simulink model "LQR"  (R2019a)
settings: Solver=FixedStepAuto  StartTime=0.0  StopTime=3  FixedStep=0.0001  RelTol=1e-3
values from neighbouring files (symbols this model uses):
  Cf = 30989    [LQR_Setup.m]
  Cr = 50154    [LQR_Setup.m]
  Iz = 111.8    [LQR_Setup.m]
  lf = 0.783    [LQR_Setup.m]
  lr = 0.752    [LQR_Setup.m]
  m = 245    [LQR_Setup.m]
undefined symbols (not defined in the file or in its folder): DiscIntNeverNeededParam, K1, K2, K3
settings Model: Creator=Johan PC  LastModifiedBy=Johan PC
settings DataIOCC: ReturnWorkspaceOutputs=off
settings DebuggingCC: ArithmeticOperatorsInVariantConditions=warning

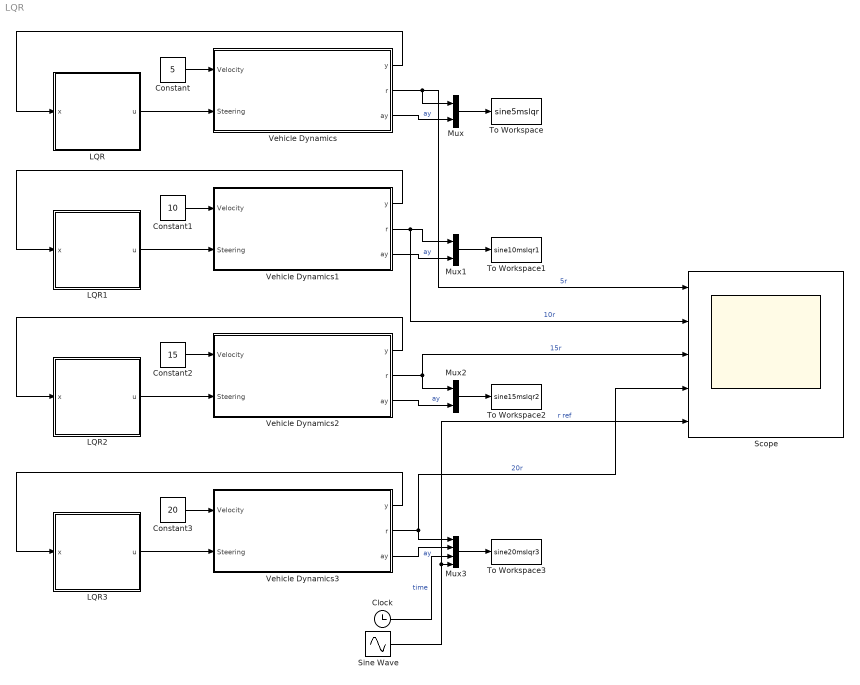
== system LQR ==
  Clock : Clock
  Constant : Constant  Value=5
  Constant1 : Constant  Value=10
  Constant2 : Constant  Value=15
  Constant3 : Constant  Value=20
  LQR : Subsystem
  LQR1 : Subsystem
  LQR2 : Subsystem
  LQR3 : Subsystem
  Mux : Mux  Inputs=2
  Mux1 : Mux  Inputs=2
  Mux2 : Mux  Inputs=2
  Mux3 : Mux
  Scope : Scope  NumInputPorts=5
  Sine Wave : Sin  Amplitude=2  Frequency=2  SampleTime=0
  To Workspace : ToWorkspace  VariableName=sine5mslqr  SampleTime=-1
      settings: Save2DSignal=2-D array (concatenate along first dimension)
  To Workspace1 : ToWorkspace  VariableName=sine10mslqr1  SampleTime=-1
      settings: Save2DSignal=2-D array (concatenate along first dimension)
  To Workspace2 : ToWorkspace  VariableName=sine15mslqr2  SampleTime=-1
      settings: Save2DSignal=2-D array (concatenate along first dimension)
  To Workspace3 : ToWorkspace  VariableName=sine20mslqr3  SampleTime=-1
      settings: Save2DSignal=2-D array (concatenate along first dimension)
  Vehicle Dynamics : Subsystem
  Vehicle Dynamics1 : Subsystem
  Vehicle Dynamics2 : Subsystem
  Vehicle Dynamics3 : Subsystem
  wires:
  Vehicle Dynamics/1("y ") -> LQR/1(x)
  LQR/1(u) -> Vehicle Dynamics/2(Steering)
  Constant/1 -> Vehicle Dynamics/1(Velocity)
  Vehicle Dynamics/2("r ") -> Scope/1, Mux/1  "5r"
  Vehicle Dynamics/3(ay) -> Mux/2  "ay"
  Mux/1 -> To Workspace/1
  Constant1/1 -> Vehicle Dynamics1/1(Velocity)
  Vehicle Dynamics1/1("y ") -> LQR1/1(x)
  LQR1/1(u) -> Vehicle Dynamics1/2(Steering)
  Vehicle Dynamics1/2("r ") -> Scope/2, Mux1/1  "10r"
  Vehicle Dynamics1/3(ay) -> Mux1/2  "ay"
  Mux1/1 -> To Workspace1/1
  Constant2/1 -> Vehicle Dynamics2/1(Velocity)
  Vehicle Dynamics2/1("y ") -> LQR2/1(x)
  LQR2/1(u) -> Vehicle Dynamics2/2(Steering)
  Vehicle Dynamics2/2("r ") -> Mux2/1, Scope/3  "15r"
  Vehicle Dynamics2/3(ay) -> Mux2/2  "ay"
  Mux2/1 -> To Workspace2/1
  Constant3/1 -> Vehicle Dynamics3/1(Velocity)
  Vehicle Dynamics3/1("y ") -> LQR3/1(x)
  LQR3/1(u) -> Vehicle Dynamics3/2(Steering)
  Vehicle Dynamics3/2("r ") -> Mux3/1, Scope/4  "20r"
  Vehicle Dynamics3/3(ay) -> Mux3/2  "ay"
  Mux3/1 -> To Workspace3/1
  Clock/1 -> Mux3/3  "time"
  Sine Wave/1 -> Scope/5, Mux3/4  "r ref"

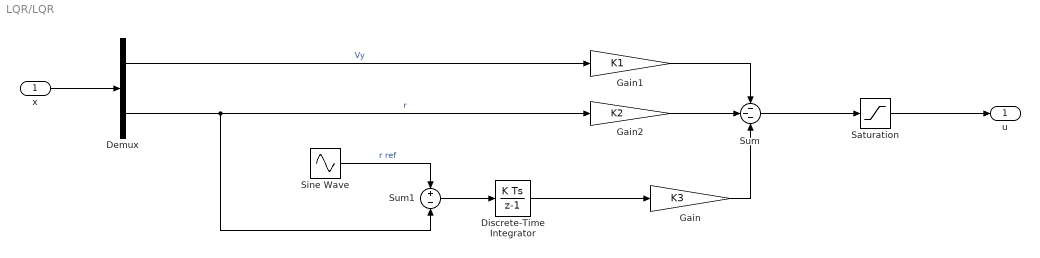
== system LQR/LQR ==
  x : Inport
  Demux : Demux  Outputs=2
  Discrete-Time Integrator : DiscreteIntegrator  SampleTime=0.001  ICPrevOutput=DiscIntNeverNeededParam  ICPrevScaledInput=DiscIntNeverNeededParam
  Gain : Gain  Gain=K3
  Gain1 : Gain  Gain=K1
  Gain2 : Gain  Gain=K2
  Saturation : Saturate  UpperLimit=0.45  LowerLimit=-0.45
  Sine Wave : Sin  Amplitude=2  Frequency=2  SampleTime=0
  Sum : Sum  Inputs=---
  Sum1 : Sum  Inputs=+-
  u : Outport
  wires:
  Discrete-Time Integrator/1 -> Gain/1
  Gain/1 -> Sum/3
  x/1 -> Demux/1
  Demux/1 -> Gain1/1  "Vy"
  Demux/2 -> Gain2/1, Sum1/2  "r"
  Gain1/1 -> Sum/1
  Gain2/1 -> Sum/2
  Sum/1 -> Saturation/1
  Sum1/1 -> Discrete-Time Integrator/1
  Sine Wave/1 -> Sum1/1  "r ref"
  Saturation/1 -> u/1

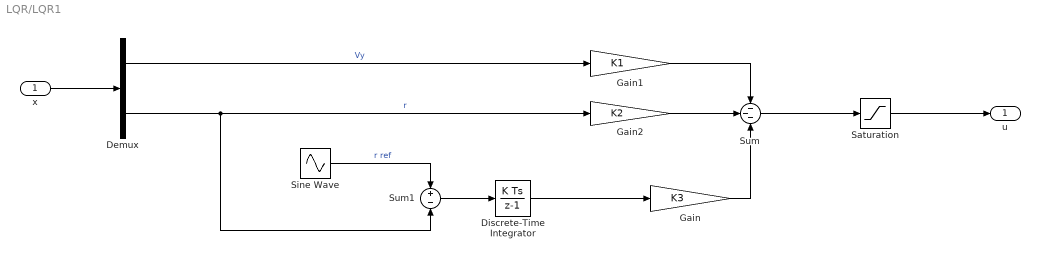
== system LQR/LQR1 ==
  x : Inport
  Demux : Demux  Outputs=2
  Discrete-Time Integrator : DiscreteIntegrator  SampleTime=0.001  ICPrevOutput=DiscIntNeverNeededParam  ICPrevScaledInput=DiscIntNeverNeededParam
  Gain : Gain  Gain=K3
  Gain1 : Gain  Gain=K1
  Gain2 : Gain  Gain=K2
  Saturation : Saturate  UpperLimit=0.45  LowerLimit=-0.45
  Sine Wave : Sin  Amplitude=2  Frequency=2  SampleTime=0
  Sum : Sum  Inputs=---
  Sum1 : Sum  Inputs=+-
  u : Outport
  wires:
  Discrete-Time Integrator/1 -> Gain/1
  Gain/1 -> Sum/3
  x/1 -> Demux/1
  Demux/1 -> Gain1/1  "Vy"
  Demux/2 -> Gain2/1, Sum1/2  "r"
  Gain1/1 -> Sum/1
  Gain2/1 -> Sum/2
  Sum/1 -> Saturation/1
  Sum1/1 -> Discrete-Time Integrator/1
  Sine Wave/1 -> Sum1/1  "r ref"
  Saturation/1 -> u/1

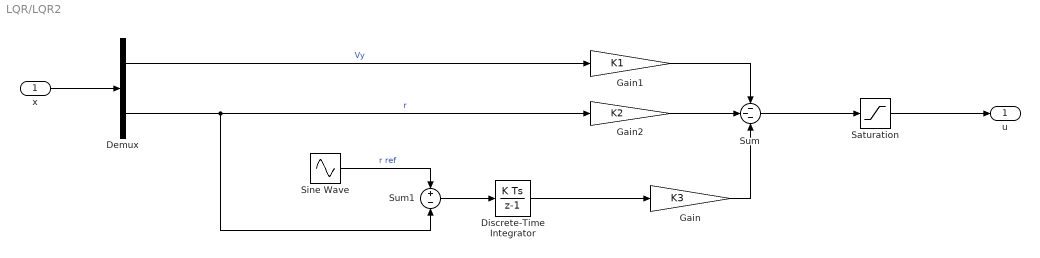
== system LQR/LQR2 ==
  x : Inport
  Demux : Demux  Outputs=2
  Discrete-Time Integrator : DiscreteIntegrator  SampleTime=0.001  ICPrevOutput=DiscIntNeverNeededParam  ICPrevScaledInput=DiscIntNeverNeededParam
  Gain : Gain  Gain=K3
  Gain1 : Gain  Gain=K1
  Gain2 : Gain  Gain=K2
  Saturation : Saturate  UpperLimit=0.45  LowerLimit=-0.45
  Sine Wave : Sin  Amplitude=2  Frequency=2  SampleTime=0
  Sum : Sum  Inputs=---
  Sum1 : Sum  Inputs=+-
  u : Outport
  wires:
  Discrete-Time Integrator/1 -> Gain/1
  Gain/1 -> Sum/3
  x/1 -> Demux/1
  Demux/1 -> Gain1/1  "Vy"
  Demux/2 -> Gain2/1, Sum1/2  "r"
  Gain1/1 -> Sum/1
  Gain2/1 -> Sum/2
  Sum/1 -> Saturation/1
  Sum1/1 -> Discrete-Time Integrator/1
  Sine Wave/1 -> Sum1/1  "r ref"
  Saturation/1 -> u/1

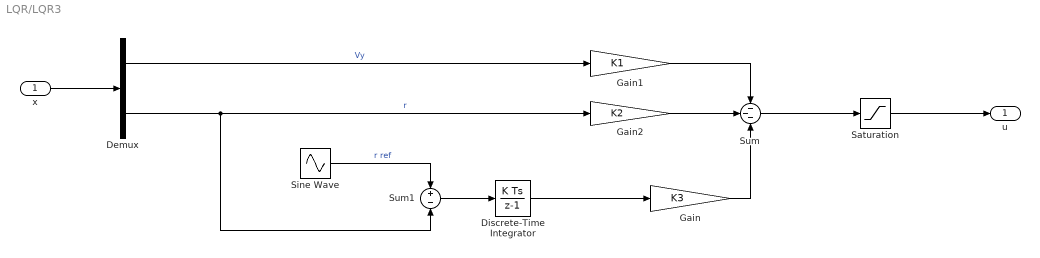
== system LQR/LQR3 ==
  x : Inport
  Demux : Demux  Outputs=2
  Discrete-Time Integrator : DiscreteIntegrator  SampleTime=0.001  ICPrevOutput=DiscIntNeverNeededParam  ICPrevScaledInput=DiscIntNeverNeededParam
  Gain : Gain  Gain=K3
  Gain1 : Gain  Gain=K1
  Gain2 : Gain  Gain=K2
  Saturation : Saturate  UpperLimit=0.45  LowerLimit=-0.45
  Sine Wave : Sin  Amplitude=2  Frequency=2  SampleTime=0
  Sum : Sum  Inputs=---
  Sum1 : Sum  Inputs=+-
  u : Outport
  wires:
  Discrete-Time Integrator/1 -> Gain/1
  Gain/1 -> Sum/3
  x/1 -> Demux/1
  Demux/1 -> Gain1/1  "Vy"
  Demux/2 -> Gain2/1, Sum1/2  "r"
  Gain1/1 -> Sum/1
  Gain2/1 -> Sum/2
  Sum/1 -> Saturation/1
  Sum1/1 -> Discrete-Time Integrator/1
  Sine Wave/1 -> Sum1/1  "r ref"
  Saturation/1 -> u/1

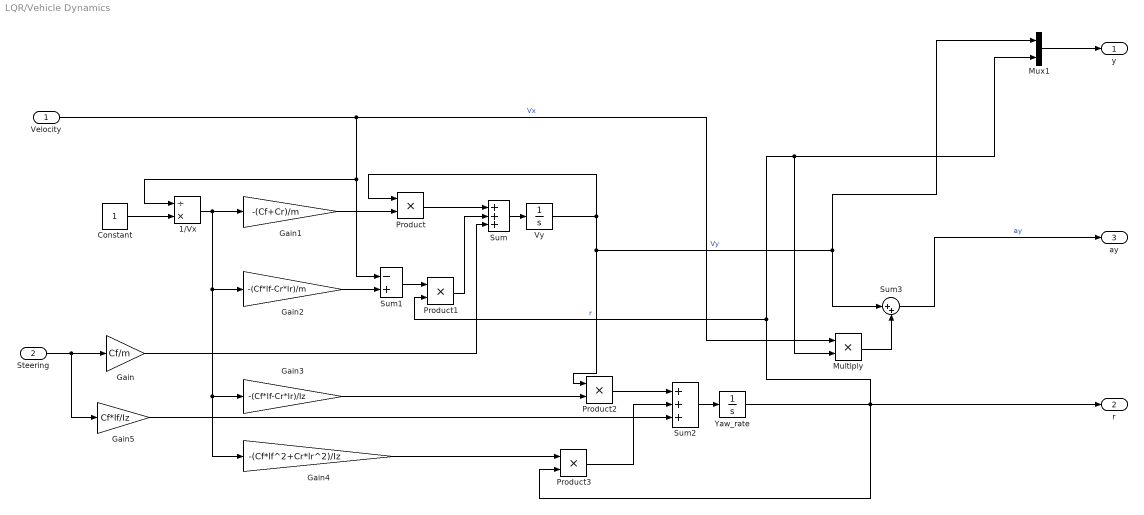
== system LQR/Vehicle Dynamics ==
  Velocity : Inport
  Steering : Inport  Port=2
  1/Vx : Product  Inputs=/*
  Constant : Constant
  Gain : Gain  Gain=Cf/m
  Gain1 : Gain  Gain=-(Cf+Cr)/m
  Gain2 : Gain  Gain=-(Cf*lf-Cr*lr)/m
  Gain3 : Gain  Gain=-(Cf*lf-Cr*lr)/Iz
  Gain4 : Gain  Gain=-(Cf*lf^2+Cr*lr^2)/Iz
  Gain5 : Gain  Gain=Cf*lf/Iz
  Multiply : Product
  Mux1 : Mux  Inputs=2
  Product{,1..3} (4 alike) : Product
  Sum : Sum  Inputs=+++
  Sum1 : Sum  Inputs=-+
  Sum2 : Sum  Inputs=+++
  Sum3 : Sum  Inputs=|++
  Vy : Integrator
  "Yaw_rate " : Integrator
  "y " : Outport
  "r " : Outport  Port=2
  ay : Outport  Port=3
  wires:
  Sum2/1 -> "Yaw_rate "/1
  Gain2/1 -> Sum1/2
  Gain4/1 -> Product3/1
  Constant/1 -> 1/Vx/2
  Gain3/1 -> Product2/2
  1/Vx/1 -> Gain4/1, Gain3/1, Gain2/1, Gain1/1
  Product2/1 -> Sum2/1
  Product3/1 -> Sum2/2
  Gain5/1 -> Sum2/3
  Sum1/1 -> Product1/1
  "Yaw_rate "/1 -> Multiply/2, Mux1/2, Product1/2, "r "/1, Product3/2  "r"
  Gain/1 -> Sum/3
  Steering/1 -> Gain/1, Gain5/1
  Gain1/1 -> Product/2
  Product/1 -> Sum/1
  Vy/1 -> Mux1/1, Sum3/1, Product2/1, Product/1  "Vy"
  Sum/1 -> Vy/1
  Velocity/1 -> Multiply/1, 1/Vx/1, Sum1/1  "Vx"
  Product1/1 -> Sum/2
  Multiply/1 -> Sum3/2
  Sum3/1 -> ay/1  "ay"
  Mux1/1 -> "y "/1

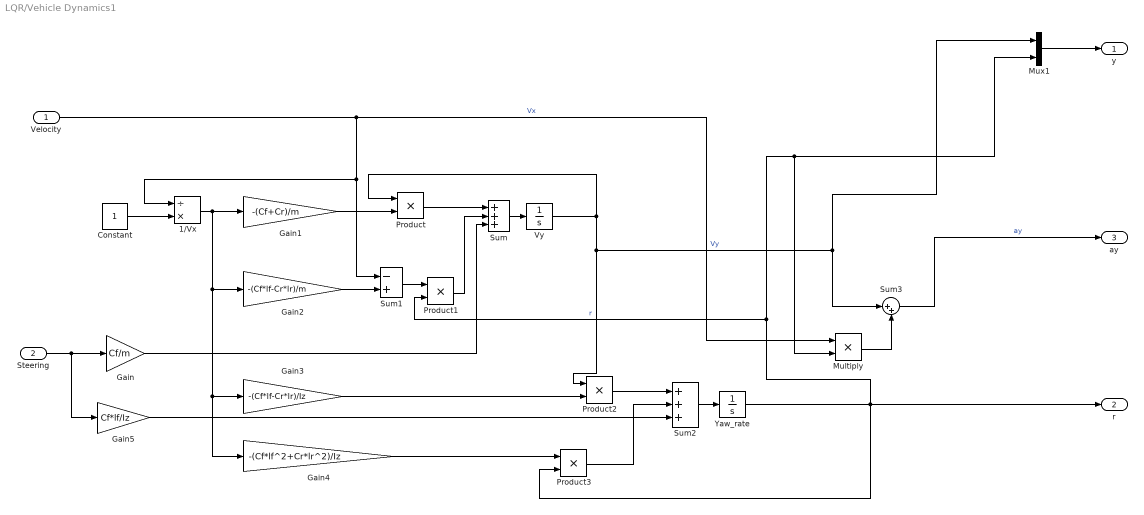
== system LQR/Vehicle Dynamics1 ==
  Velocity : Inport
  Steering : Inport  Port=2
  1/Vx : Product  Inputs=/*
  Constant : Constant
  Gain : Gain  Gain=Cf/m
  Gain1 : Gain  Gain=-(Cf+Cr)/m
  Gain2 : Gain  Gain=-(Cf*lf-Cr*lr)/m
  Gain3 : Gain  Gain=-(Cf*lf-Cr*lr)/Iz
  Gain4 : Gain  Gain=-(Cf*lf^2+Cr*lr^2)/Iz
  Gain5 : Gain  Gain=Cf*lf/Iz
  Multiply : Product
  Mux1 : Mux  Inputs=2
  Product{,1..3} (4 alike) : Product
  Sum : Sum  Inputs=+++
  Sum1 : Sum  Inputs=-+
  Sum2 : Sum  Inputs=+++
  Sum3 : Sum  Inputs=|++
  Vy : Integrator
  "Yaw_rate " : Integrator
  "y " : Outport
  "r " : Outport  Port=2
  ay : Outport  Port=3
  wires:
  Sum2/1 -> "Yaw_rate "/1
  Gain2/1 -> Sum1/2
  Gain4/1 -> Product3/1
  Constant/1 -> 1/Vx/2
  Gain3/1 -> Product2/2
  1/Vx/1 -> Gain4/1, Gain3/1, Gain2/1, Gain1/1
  Product2/1 -> Sum2/1
  Product3/1 -> Sum2/2
  Gain5/1 -> Sum2/3
  Sum1/1 -> Product1/1
  "Yaw_rate "/1 -> Multiply/2, Mux1/2, Product1/2, "r "/1, Product3/2  "r"
  Gain/1 -> Sum/3
  Steering/1 -> Gain/1, Gain5/1
  Gain1/1 -> Product/2
  Product/1 -> Sum/1
  Vy/1 -> Mux1/1, Sum3/1, Product2/1, Product/1  "Vy"
  Sum/1 -> Vy/1
  Velocity/1 -> Multiply/1, 1/Vx/1, Sum1/1  "Vx"
  Product1/1 -> Sum/2
  Multiply/1 -> Sum3/2
  Sum3/1 -> ay/1  "ay"
  Mux1/1 -> "y "/1

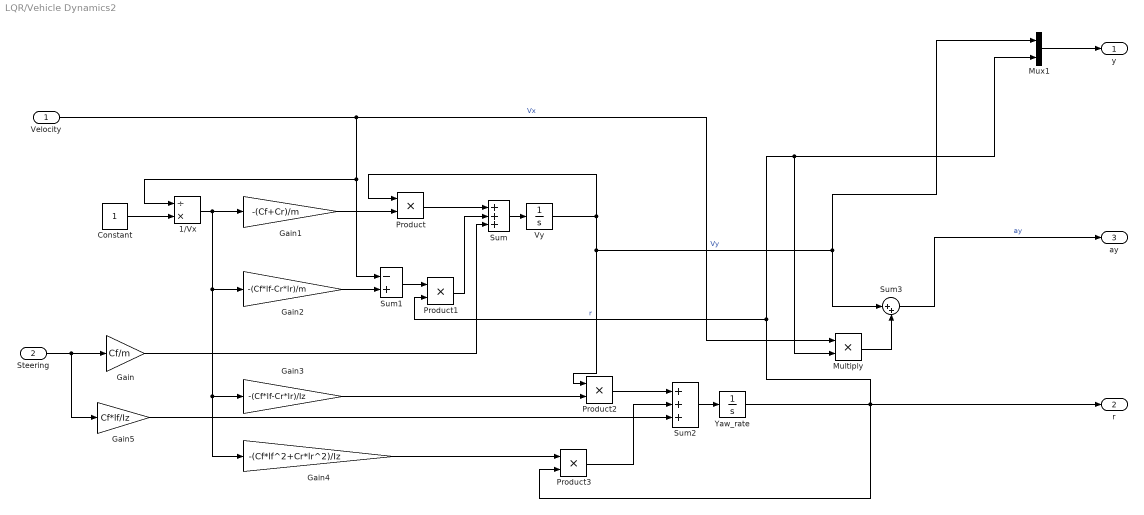
== system LQR/Vehicle Dynamics2 ==
  Velocity : Inport
  Steering : Inport  Port=2
  1/Vx : Product  Inputs=/*
  Constant : Constant
  Gain : Gain  Gain=Cf/m
  Gain1 : Gain  Gain=-(Cf+Cr)/m
  Gain2 : Gain  Gain=-(Cf*lf-Cr*lr)/m
  Gain3 : Gain  Gain=-(Cf*lf-Cr*lr)/Iz
  Gain4 : Gain  Gain=-(Cf*lf^2+Cr*lr^2)/Iz
  Gain5 : Gain  Gain=Cf*lf/Iz
  Multiply : Product
  Mux1 : Mux  Inputs=2
  Product{,1..3} (4 alike) : Product
  Sum : Sum  Inputs=+++
  Sum1 : Sum  Inputs=-+
  Sum2 : Sum  Inputs=+++
  Sum3 : Sum  Inputs=|++
  Vy : Integrator
  "Yaw_rate " : Integrator
  "y " : Outport
  "r " : Outport  Port=2
  ay : Outport  Port=3
  wires:
  Sum2/1 -> "Yaw_rate "/1
  Gain2/1 -> Sum1/2
  Gain4/1 -> Product3/1
  Constant/1 -> 1/Vx/2
  Gain3/1 -> Product2/2
  1/Vx/1 -> Gain4/1, Gain3/1, Gain2/1, Gain1/1
  Product2/1 -> Sum2/1
  Product3/1 -> Sum2/2
  Gain5/1 -> Sum2/3
  Sum1/1 -> Product1/1
  "Yaw_rate "/1 -> Multiply/2, Mux1/2, Product1/2, "r "/1, Product3/2  "r"
  Gain/1 -> Sum/3
  Steering/1 -> Gain/1, Gain5/1
  Gain1/1 -> Product/2
  Product/1 -> Sum/1
  Vy/1 -> Mux1/1, Sum3/1, Product2/1, Product/1  "Vy"
  Sum/1 -> Vy/1
  Velocity/1 -> Multiply/1, 1/Vx/1, Sum1/1  "Vx"
  Product1/1 -> Sum/2
  Multiply/1 -> Sum3/2
  Sum3/1 -> ay/1  "ay"
  Mux1/1 -> "y "/1

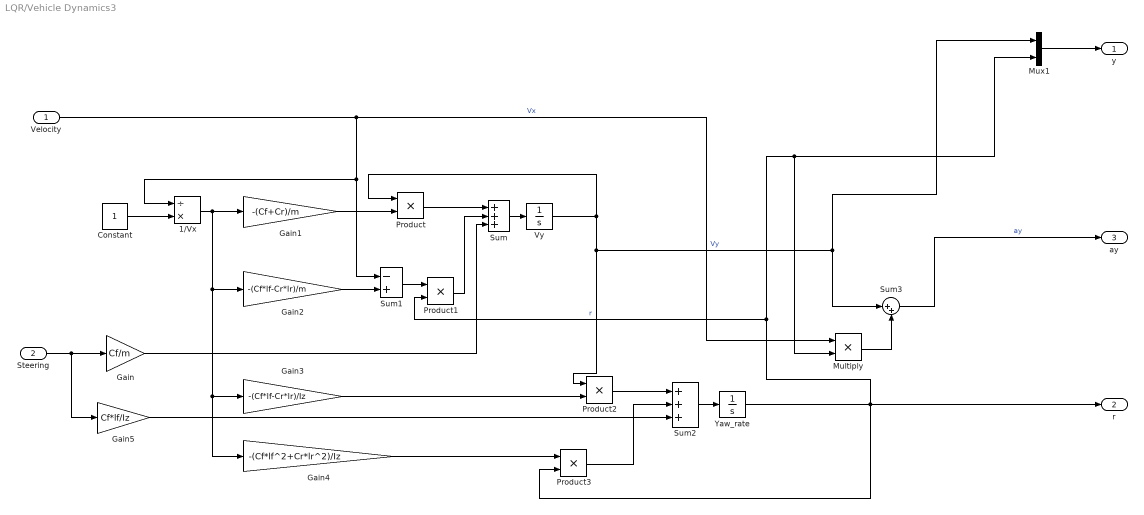
== system LQR/Vehicle Dynamics3 ==
  Velocity : Inport
  Steering : Inport  Port=2
  1/Vx : Product  Inputs=/*
  Constant : Constant
  Gain : Gain  Gain=Cf/m
  Gain1 : Gain  Gain=-(Cf+Cr)/m
  Gain2 : Gain  Gain=-(Cf*lf-Cr*lr)/m
  Gain3 : Gain  Gain=-(Cf*lf-Cr*lr)/Iz
  Gain4 : Gain  Gain=-(Cf*lf^2+Cr*lr^2)/Iz
  Gain5 : Gain  Gain=Cf*lf/Iz
  Multiply : Product
  Mux1 : Mux  Inputs=2
  Product{,1..3} (4 alike) : Product
  Sum : Sum  Inputs=+++
  Sum1 : Sum  Inputs=-+
  Sum2 : Sum  Inputs=+++
  Sum3 : Sum  Inputs=|++
  Vy : Integrator
  "Yaw_rate " : Integrator
  "y " : Outport
  "r " : Outport  Port=2
  ay : Outport  Port=3
  wires:
  Sum2/1 -> "Yaw_rate "/1
  Gain2/1 -> Sum1/2
  Gain4/1 -> Product3/1
  Constant/1 -> 1/Vx/2
  Gain3/1 -> Product2/2
  1/Vx/1 -> Gain4/1, Gain3/1, Gain2/1, Gain1/1
  Product2/1 -> Sum2/1
  Product3/1 -> Sum2/2
  Gain5/1 -> Sum2/3
  Sum1/1 -> Product1/1
  "Yaw_rate "/1 -> Multiply/2, Mux1/2, Product1/2, "r "/1, Product3/2  "r"
  Gain/1 -> Sum/3
  Steering/1 -> Gain/1, Gain5/1
  Gain1/1 -> Product/2
  Product/1 -> Sum/1
  Vy/1 -> Mux1/1, Sum3/1, Product2/1, Product/1  "Vy"
  Sum/1 -> Vy/1
  Velocity/1 -> Multiply/1, 1/Vx/1, Sum1/1  "Vx"
  Product1/1 -> Sum/2
  Multiply/1 -> Sum3/2
  Sum3/1 -> ay/1  "ay"
  Mux1/1 -> "y "/1
